simulink model "motorul"  (R2023b)
settings: Solver=VariableStepAuto  StartTime=0.0  StopTime=10.0  RelTol=1e-3
settings Model: Creator=diana.forrai  LastModifiedBy=diana.forrai

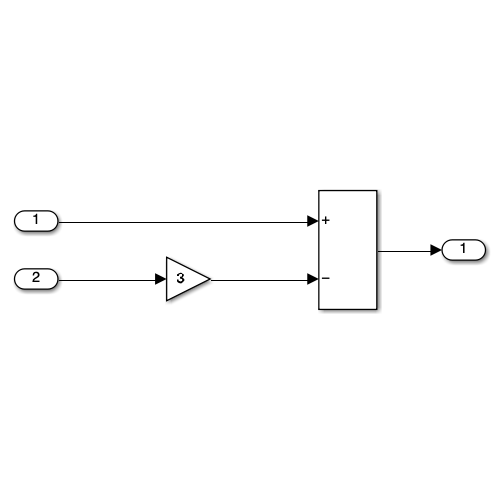
[thumbnail: Simulink's stored preview of the top-level diagram]
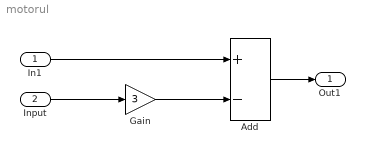
== system motorul ==
  In1 : Inport
  Input : Inport  Port=2
  Add : Sum  Inputs=+-
  Gain : Gain  Gain=3
  Out1 : Outport
  wires:
  Add/1 -> Out1/1
  In1/1 -> Add/1
  Input/1 -> Gain/1
  Gain/1 -> Add/2
